simulink model "Project2_Tweedle"  (R2017a)
settings: Solver=ode4  StartTime=0.0  StopTime=5*T  FixedStep=dt  RelTol=1e-3  EnableMultiTasking=on
values from neighbouring files (symbols this model uses):
  CLVD = .0146    (= 0.0146)    [parameters_SA_LV_Tweedle.m]
  CLVS = .00003    (= 3e-05)    [parameters_SA_LV_Tweedle.m]
  Csa = .00175    (= 0.00175)    [parameters_SA_LV_Tweedle.m]
  Pla = 5    [parameters_SA_LV_Tweedle.m]
  Plvi = 5    [parameters_SA_LV_Tweedle.m]
  Psai = 80    [parameters_SA_LV_Tweedle.m]
  RAo = 0.01    [parameters_SA_LV_Tweedle.m]
  Rmi = 0.01    [parameters_SA_LV_Tweedle.m]
  Rs = 17.86    [parameters_SA_LV_Tweedle.m]
  T = 0.0125    [parameters_SA_LV_Tweedle.m]
  tauD = .001    (= 0.001)    [parameters_SA_LV_Tweedle.m]
  tauS = .0025    (= 0.0025)    [parameters_SA_LV_Tweedle.m]
  Ts = 0.0050    (= 0.005)    [parameters_SA_LV_Tweedle.m]
  Vlvd = .027    (= 0.027)    [parameters_SA_LV_Tweedle.m]
  Vsad = .825    (= 0.825)    [parameters_SA_LV_Tweedle.m]
settings Model: Creator=Jake Tweedle  LastModifiedBy=Jake Tweedle

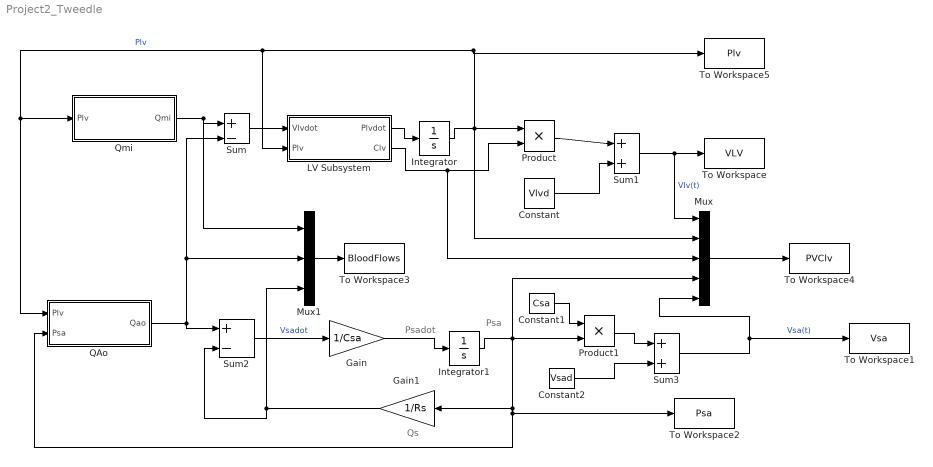
== system Project2_Tweedle ==
  note: Qs
  note: Psa
  note: Psadot
  Constant : Constant  Value=Vlvd
  Constant1 : Constant  Value=Csa
  Constant2 : Constant  Value=Vsad
  Gain : Gain  Gain=1/Csa
  Gain1 : Gain  Gain=1/Rs
  Integrator : Integrator  InitialCondition=Plvi
  Integrator1 : Integrator  InitialCondition=Psai
  LV Subsystem : Subsystem
  Mux : Mux  Inputs=5
  Mux1 : Mux  Inputs=3
  Product : Product
  Product1 : Product
  QAo : Subsystem
  Qmi : Subsystem
  Sum : Sum  Inputs=+|-
  Sum1 : Sum  Inputs=+||+
  Sum2 : Sum  Inputs=+||-
  Sum3 : Sum  Inputs=+||+
  To Workspace : ToWorkspace  VariableName=VLV  SaveFormat=Timeseries  SampleTime=-1
  To Workspace1 : ToWorkspace  VariableName=Vsa  SaveFormat=Timeseries  SampleTime=-1
  To Workspace2 : ToWorkspace  VariableName=Psa  SaveFormat=Timeseries  SampleTime=-1
  To Workspace3 : ToWorkspace  VariableName=BloodFlows  SaveFormat=Structure With Time  SampleTime=-1
  To Workspace4 : ToWorkspace  VariableName=PVClv  SaveFormat=Structure With Time  SampleTime=-1
  To Workspace5 : ToWorkspace  VariableName=Plv  SaveFormat=Timeseries  SampleTime=-1
  wires:
  Qmi/1(Qmi) -> Mux1/1, Sum/1
  Sum/1 -> LV Subsystem/1(Vlvdot)
  LV Subsystem/1(Plvdot) -> Integrator/1
  LV Subsystem/2(Clv) -> Mux/3, Product/2
  Product/1 -> Sum1/1
  Constant/1 -> Sum1/2
  Sum1/1 -> Mux/1, To Workspace/1  "Vlv(t)"
  QAo/1(Qao) -> Sum2/1, Mux1/2, Sum/2
  Sum2/1 -> Gain/1  "Vsadot"
  Gain/1 -> Integrator1/1
  Integrator1/1 -> Product1/2, QAo/2(Psa), To Workspace2/1, Gain1/1, Mux/4
  Sum3/1 -> To Workspace1/1, Mux/5  "Vsa(t)"
  Gain1/1 -> Sum2/2, Mux1/3
  Mux1/1 -> To Workspace3/1
  Integrator/1 -> Mux/2, To Workspace5/1, LV Subsystem/2(Plv), Qmi/1(Plv), QAo/1(Plv), Product/1  "Plv"
  Mux/1 -> To Workspace4/1
  Constant1/1 -> Product1/1
  Product1/1 -> Sum3/1
  Constant2/1 -> Sum3/2

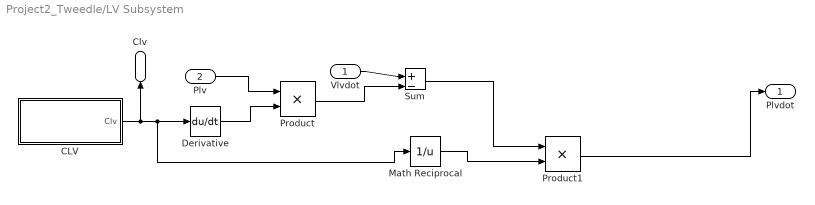
== system Project2_Tweedle/LV Subsystem ==
  Vlvdot : Inport
  Plv : Inport  Port=2
  CLV : Subsystem
  Derivative : Derivative
  Math Reciprocal : Math  Operator=reciprocal  SaturateOnIntegerOverflow=on
  Product : Product
  Product1 : Product
  Sum : Sum  Inputs=+||-
  Plvdot : Outport
  Clv : Outport  Port=2
  wires:
  Derivative/1 -> Product/2
  Plv/1 -> Product/1
  Vlvdot/1 -> Sum/1
  Product/1 -> Sum/2
  Sum/1 -> Product1/1
  CLV/1(Clv) -> Clv/1, Math Reciprocal/1, Derivative/1
  Math Reciprocal/1 -> Product1/2
  Product1/1 -> Plvdot/1

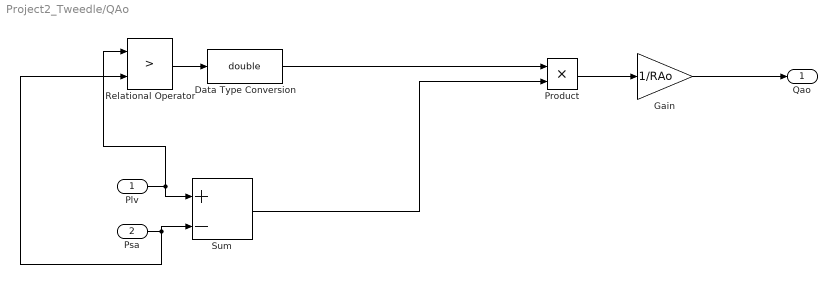
== system Project2_Tweedle/QAo ==
  Plv : Inport
  Psa : Inport  Port=2
  Data Type Conversion : DataTypeConversion  OutDataTypeStr=double
  Gain : Gain  Gain=1/RAo
  Product : Product
  Relational Operator : RelationalOperator  Operator=>  OutDataTypeStr=boolean  RndMeth=Simplest
  Sum : Sum  Inputs=+||-
  Qao : Outport
  wires:
  Plv/1 -> Relational Operator/1, Sum/1
  Psa/1 -> Sum/2, Relational Operator/2
  Relational Operator/1 -> Data Type Conversion/1
  Data Type Conversion/1 -> Product/1
  Sum/1 -> Product/2
  Product/1 -> Gain/1
  Gain/1 -> Qao/1

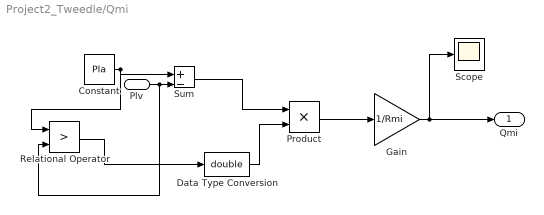
== system Project2_Tweedle/Qmi ==
  Plv : Inport
  Constant : Constant  Value=Pla
  Data Type Conversion : DataTypeConversion  OutDataTypeStr=double
  Gain : Gain  Gain=1/Rmi
  Product : Product
  Relational Operator : RelationalOperator  Operator=>  OutDataTypeStr=boolean  RndMeth=Simplest
  Scope : Scope
  Sum : Sum  Inputs=+||-
  Qmi : Outport
  wires:
  Constant/1 -> Relational Operator/1, Sum/1
  Gain/1 -> Scope/1, Qmi/1
  Relational Operator/1 -> Data Type Conversion/1
  Product/1 -> Gain/1
  Sum/1 -> Product/1
  Data Type Conversion/1 -> Product/2
  Plv/1 -> Relational Operator/2, Sum/2

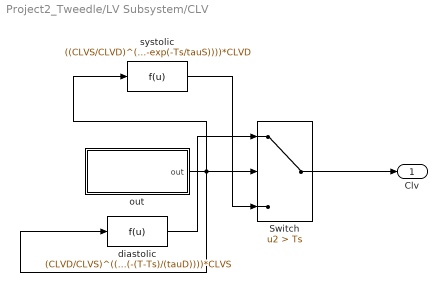
== system Project2_Tweedle/LV Subsystem/CLV ==
  Switch : Switch  Criteria=u2 > Threshold  Threshold=Ts
  diastolic : Fcn  Expr=(CLVD/CLVS)^((1-exp(-(u-Ts)/(tauD)))/(1-exp(-(T-Ts)/(tauD))))*CLVS
  out : Subsystem
  systolic : Fcn  Expr=((CLVS/CLVD)^((1-exp(-u/tauS))/(1-exp(-Ts/tauS))))*CLVD
  Clv : Outport
  wires:
  out/1(out) -> diastolic/1, Switch/2, systolic/1
  Switch/1 -> Clv/1
  diastolic/1 -> Switch/1
  systolic/1 -> Switch/3

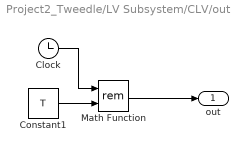
== system Project2_Tweedle/LV Subsystem/CLV/out ==
  Clock : Clock
  Constant1 : Constant  Value=T
  Math Function : Math  Operator=rem  SaturateOnIntegerOverflow=on
  out : Outport
  wires:
  Constant1/1 -> Math Function/2
  Clock/1 -> Math Function/1
  Math Function/1 -> out/1
